simulink library "MATLAB_Function_lib"  (R2017b)
settings: Solver=VariableStepAuto  StartTime=0.0  StopTime=10.0  RelTol=1e-3
undefined symbols (not defined in the file or in its folder): Newton, Raphson
libraries: simulink x1
(part 1 of 3)
settings Model: Creator=ktrinh  LastModifiedBy=hbourbou

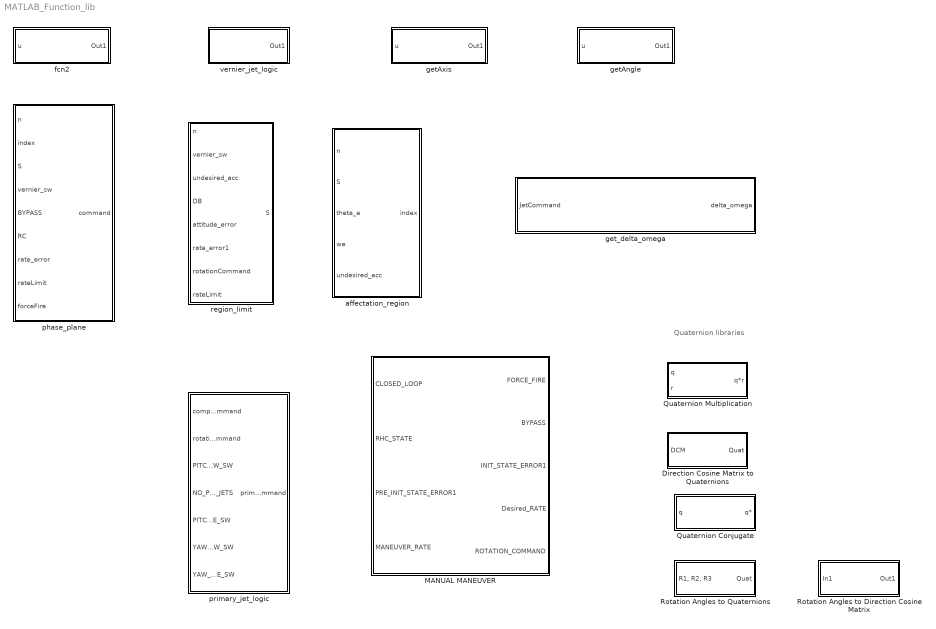
== system MATLAB_Function_lib ==
  note: Quaternion libraries
  Direction Cosine Matrix to Quaternions : Subsystem
  MANUAL MANEUVER : Subsystem
  Quaternion Conjugate : Subsystem
  Quaternion Multiplication : Subsystem
  Rotation Angles to Direction Cosine Matrix : Subsystem
  Rotation Angles to Quaternions : Subsystem
  affectation_region : Subsystem
  fcn2 : Subsystem
  getAngle : Subsystem
  getAxis : Subsystem
  get_delta_omega : Subsystem
  phase_plane : Subsystem
  primary_jet_logic : Subsystem
  region_limit : Subsystem
  vernier_jet_logic : Subsystem

== system MATLAB_Function_lib/Direction Cosine Matrix to Quaternions ==
  DCM : Inport  Unit=1  PortDimensions=[3,3]
  If : If
  Merge : Merge  InitialOutput=[1 0 0 0]
  Negative Trace : Subsystem
  Positive Trace : Subsystem  TreatAsAtomicUnit=on
  "Reshape 3x3 -> 9" : Reshape  OutputDimensions=[9,1]
  trace(DCM) : Subsystem
  Quat : Outport  Unit=1  PortDimensions=4
  wires:
  If/1 -> Positive Trace/Action
  Positive Trace/1(qw qx qy qz) -> Merge/1
  trace(DCM)/1(trace(DCM)) -> Positive Trace/1(trace(DCM)), If/1
  DCM/1 -> "Reshape 3x3 -> 9"/1
  "Reshape 3x3 -> 9"/1 -> trace(DCM)/1(DCM), Negative Trace/1(DCM), Positive Trace/2(DCM)
  Negative Trace/1(qw qx qy qz) -> Merge/2
  Merge/1 -> Quat/1
  If/2 -> Negative Trace/Action

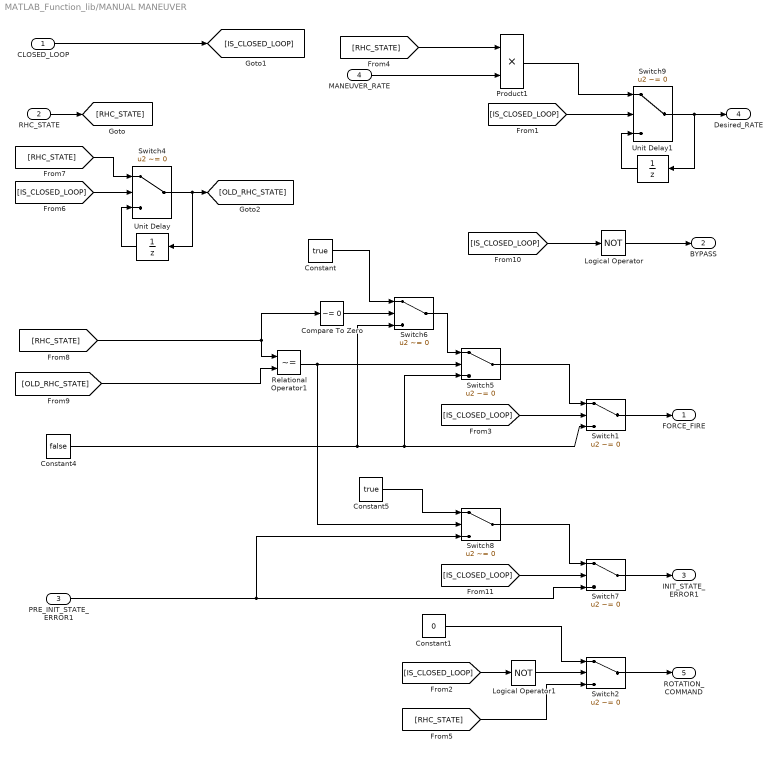
== system MATLAB_Function_lib/MANUAL MANEUVER ==
  CLOSED_LOOP : Inport
  RHC_STATE : Inport  Port=2
  PRE_INIT_STATE_ERROR1 : Inport  Port=3
  MANEUVER_RATE : Inport  Port=4
  Compare To Zero : simulink/Logic and Bit Operations/Compare To Zero  relop=~=  OutDataTypeStr=boolean
  Constant : Constant  Value=true
  Constant1 : Constant  Value=0
  Constant4 : Constant  Value=false
  Constant5 : Constant  Value=true
  Logical Operator : Logic  Operator=NOT  AllPortsSameDT=off  OutDataTypeStr=boolean
  Logical Operator1 : Logic  Operator=NOT  AllPortsSameDT=off  OutDataTypeStr=boolean
  Product1 : Product
  Relational Operator1 : RelationalOperator  Operator=~=  OutDataTypeStr=boolean  RndMeth=Simplest
  Switch{1..2,4..9} (8 alike) : Switch  Criteria=u2 ~= 0
  Unit Delay : UnitDelay  SampleTime=-1
  Unit Delay1 : UnitDelay  SampleTime=-1
  FORCE_FIRE : Outport
  BYPASS : Outport  Port=2
  INIT_STATE_ERROR1 : Outport  Port=3
  Desired_RATE : Outport  Port=4
  ROTATION_COMMAND : Outport  Port=5
  wires:
  Constant4/1 -> Switch6/3, Switch5/3, Switch1/3
  Switch1/1 -> FORCE_FIRE/1
  CLOSED_LOOP/1 -> [IS_CLOSED_LOOP]
  [IS_CLOSED_LOOP] -> Switch1/2
  RHC_STATE/1 -> [RHC_STATE]
  Switch4/1 -> Unit Delay/1, [OLD_RHC_STATE]
  [IS_CLOSED_LOOP] -> Switch4/2
  [RHC_STATE] -> Switch4/1
  Unit Delay/1 -> Switch4/3
  Switch5/1 -> Switch1/1
  [RHC_STATE] -> Compare To Zero/1, Relational Operator1/1
  [OLD_RHC_STATE] -> Relational Operator1/2
  Switch6/1 -> Switch5/1
  Compare To Zero/1 -> Switch6/2
  Constant/1 -> Switch6/1
  Logical Operator/1 -> BYPASS/1
  [IS_CLOSED_LOOP] -> Logical Operator/1
  Switch7/1 -> INIT_STATE_ERROR1/1
  Switch8/1 -> Switch7/1
  [IS_CLOSED_LOOP] -> Switch7/2
  Constant5/1 -> Switch8/1
  Relational Operator1/1 -> Switch8/2, Switch5/2
  PRE_INIT_STATE_ERROR1/1 -> Switch8/3, Switch7/3
  Switch9/1 -> Unit Delay1/1, Desired_RATE/1
  Product1/1 -> Switch9/1
  [IS_CLOSED_LOOP] -> Switch9/2
  [RHC_STATE] -> Product1/1
  MANEUVER_RATE/1 -> Product1/2
  Unit Delay1/1 -> Switch9/3
  [RHC_STATE] -> Switch2/3
  [IS_CLOSED_LOOP] -> Logical Operator1/1
  Constant1/1 -> Switch2/1
  Switch2/1 -> ROTATION_COMMAND/1
  Logical Operator1/1 -> Switch2/2

== system MATLAB_Function_lib/Quaternion Conjugate ==
  q : Inport  Unit=1
  Demux : Demux
  Mux : Mux
  Unary Minus : UnaryMinus
  Unary Minus1 : UnaryMinus
  Unary Minus2 : UnaryMinus
  q* : Outport  Unit=1
  wires:
  Mux/1 -> q*/1
  Demux/2 -> Unary Minus/1
  Unary Minus1/1 -> Mux/3
  Demux/4 -> Unary Minus2/1
  Demux/1 -> Mux/1
  Unary Minus/1 -> Mux/2
  Demux/3 -> Unary Minus1/1
  Unary Minus2/1 -> Mux/4
  q/1 -> Demux/1

== system MATLAB_Function_lib/Quaternion Multiplication ==
  q : Inport  Unit=1
  r : Inport  Port=2  Unit=1
  Mux : Mux
  q0 : Subsystem
  q1 : Subsystem
  q2 : Subsystem
  q3 : Subsystem
  q*r : Outport  Unit=1
  wires:
  q/1 -> q3/1(q), q2/1(q), q1/1(q), q0/1(q)
  q1/1(q1) -> Mux/2
  q0/1(q0) -> Mux/1
  q2/1(q2) -> Mux/3
  r/1 -> q3/2(r), q2/2(r), q1/2(r), q0/2(r)
  Mux/1 -> q*r/1
  q3/1(q3) -> Mux/4

== system MATLAB_Function_lib/Rotation Angles to Direction Cosine Matrix ==
  In1 : Inport  Unit=rad  PortDimensions=3
  Create 3x3 Matrix : Subsystem  mask(Create 3x3 Matrix){}
      mask help: shared_aeroblks:sharedaeroblkutil:blockCreate3x3MatrixDesc
      mask init:
      | if license('test','aerospace_blockset')
      |     aerosharedicon('shared');
      | elseif license('test','powertrain_blockset')
      |     sharedautoicon('shared');
      | end
      mask Help: eval('if license(''test'',''aerospace_blockset'')aerosharedhelp(''create_threebythree_matrix'');elseif license(''test'',''powertrain_blockset'')sharedautohelp(''create_threebythree_matrix'');end')
      mask Display:
      | port_label('input',1,'A_{11}','texmode','on');
      | port_label('input',2,'A_{12}','texmode','on');
      | port_label('input',3,'A_{13}','texmode','on');
      | port_label('input',4,'A_{21}','texmode','on');
      | port_label('input',5,'A_{22}','texmode','on');
      | port_label('input',6,'A_{23}','texmode','on');
      | port_label('input',7,'A_{31}','texmode','on');
      | port_label('input',8,'A_{32}','texmode','on');
      | port_label('input',9,'A_{33}','texmode','on');
      | port_label('output',1,'A','texmode','on');
  Fcn11 : Fcn  Expr=u(5)*u(6)
  Fcn12 : Fcn  Expr=u(1)*u(2)*u(6) + u(4)*u(3)
  Fcn13 : Fcn  Expr=-u(4)*u(2)*u(6) + u(1)*u(3)
  Fcn21 : Fcn  Expr=-u(5)*u(3)
  Fcn22 : Fcn  Expr=-u(1)*u(2)*u(3) + u(4)*u(6)
  Fcn23 : Fcn  Expr=u(4)*u(2)*u(3) + u(1)*u(6)
  Fcn31 : Fcn  Expr=u(2)
  Fcn32 : Fcn  Expr=-u(1)*u(5)
  Fcn33 : Fcn  Expr=u(4)*u(5)
  Mux : Mux  Inputs=2
  sincos : Trigonometry  Operator=sincos
  Out1 : Outport  Unit=1  PortDimensions=[3,3]
  wires:
  sincos/2 -> Mux/2
  Create 3x3 Matrix/1(Matrix) -> Out1/1
  Fcn11/1 -> Create 3x3 Matrix/1(M11)
  In1/1 -> sincos/1
  Fcn31/1 -> Create 3x3 Matrix/7(M31)
  Fcn22/1 -> Create 3x3 Matrix/5(M22)
  Fcn21/1 -> Create 3x3 Matrix/4(M21)
  Fcn23/1 -> Create 3x3 Matrix/6(M23)
  Fcn33/1 -> Create 3x3 Matrix/9(M33)
  Mux/1 -> Fcn11/1, Fcn12/1, Fcn13/1, Fcn21/1, Fcn32/1, Fcn33/1, Fcn31/1, Fcn23/1, Fcn22/1
  Fcn13/1 -> Create 3x3 Matrix/3(M13)
  sincos/1 -> Mux/1
  Fcn12/1 -> Create 3x3 Matrix/2(M12)
  Fcn32/1 -> Create 3x3 Matrix/8(M32)

== system MATLAB_Function_lib/Rotation Angles to Quaternions ==
  "R1, R2, R3" : Inport  Unit=rad
  1/2 : Gain  Gain=0.5  SaturateOnIntegerOverflow=on  OutDataTypeStr=Inherit: Same as input  ParamDataTypeStr=Inherit: Same as input
  Mux1 : Mux  Inputs=2
  Mux2 : Mux
  q0 : Fcn  Expr=u(4)*u(5)*u(6) - u(1)*u(2)*u(3)
  q1 : Fcn  Expr=u(4)*u(2)*u(3) + u(1)*u(5)*u(6)
  q2 : Fcn  Expr=u(4)*u(2)*u(6) - u(1)*u(5)*u(3)
  q3 : Fcn  Expr=u(4)*u(5)*u(3) + u(1)*u(2)*u(6)
  sincos : Trigonometry  Operator=sincos
  Quat : Outport  Unit=1  InitialOutput=0
  wires:
  q1/1 -> Mux2/2
  Mux2/1 -> Quat/1
  1/2/1 -> sincos/1
  sincos/1 -> Mux1/1
  q3/1 -> Mux2/4
  Mux1/1 -> q0/1, q1/1, q2/1, q3/1
  q0/1 -> Mux2/1
  "R1, R2, R3"/1 -> 1/2/1
  sincos/2 -> Mux1/2
  q2/1 -> Mux2/3

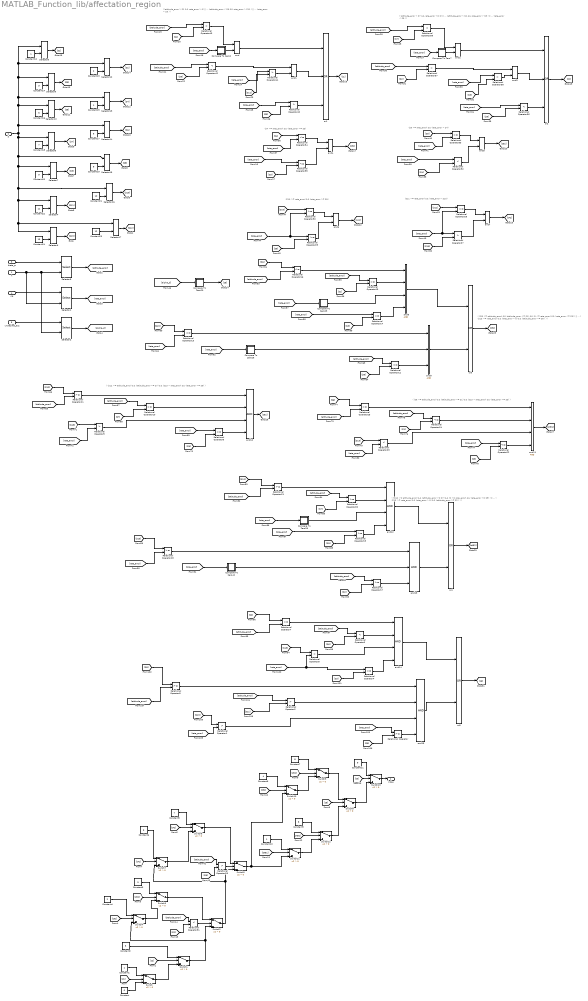
== system MATLAB_Function_lib/affectation_region ==
  note: ( (attitude_error > S1 && rate_error > 0) || ... (attitude_error < S8 && rate_error > S11 ) || ... (rate_error > S3 ) )
  note: ( (attitude_error < S7 && rate_error <= 0) || ... (attitude_error < S2 && rate_error > S5 ) || ... (rate_error < S9 ) )
  note: (S4 <= rate_error) && (rate_error <= S3)
  note: (S5 <= rate_error) && (rate_error < S4)
  note: (S10 >= rate_error) && (rate_error >= S9)
  note: (S11 >= rate_error) && (rate_error > S10)
  note: ( (S6 <= attitude_error) && (attitude_error <= S1) && (S13 < rate_error) && (rate_error <= S3) )
  note: ( ((S12 >= attitude_error) && (attitude_error >= S7) && (0 >= rate_error) && (rate_error >= S9) ) || ... ( (S13 >= rate_error) && (rate_error > 0) && (attitude_error >= S2 ) ) )
  note: ( (S12 >= attitude_error) && (attitude_error >= S7) && (S13 > rate_error) && (rate_error >= S9) )
  note: ( ((S6 <= attitude_error) && (attitude_error <= S1) && (0 <= rate_error) && (rate_error <= S3) ) || ... ( (S13 <= rate_error) && (rate_error < 0) && (attitude_error <= S8 ) ) )
  n : Inport
  S : Inport  Port=2
  theta_e : Inport  Port=3
  we : Inport  Port=4
  undesired_acc : Inport  Port=5
  Compare To Zero2 : Subsystem  mask(Compare To Zero){relop=>, OutDataTypeStr=boolean, ZeroCross=on}
      mask prompts: relop "Simulink:masks:Operator_MP"; OutDataTypeStr "Simulink:masks:OutputDataType_MP"; ZeroCross "Simulink:masks:EnableZerocrossingDetection_MP"
      mask help: Simulink:masks:CompareToZero_MD
      mask init:
      | blkName = gcb;
      | 
      | if strcmp(get_param(gcbh,'OutDataTypeStr'),'boolean')
      | 	setValue = 'boolean';
      | else
      |     setValue = 'fixdt(0, 8)';
      | end
      | 
      | set_param([blkName,'/Compare'],'relop',relop, ...
      | 	'OutDataTypeStr', setValue, 'ZeroCross', ZeroCross);
      mask TypeOptions relop: == | ~= | < | <= | >= | >
      mask TypeOptions OutDataTypeStr: Simulink:masks:uint8 | Simulink:masks:boolean
      mask Callback ZeroCross: sl('zeroCrossEnable', gcbh);
      mask Display: disp([relop,' 0'])
  Compare To Zero20 : Subsystem  mask(Compare To Zero){relop=>=, OutDataTypeStr=boolean, ZeroCross=on}
      mask prompts: relop "Simulink:masks:Operator_MP"; OutDataTypeStr "Simulink:masks:OutputDataType_MP"; ZeroCross "Simulink:masks:EnableZerocrossingDetection_MP"
      mask help: Simulink:masks:CompareToZero_MD
      mask init: same as MATLAB_Function_lib/affectation_region/Compare To Zero2
      mask TypeOptions relop: == | ~= | < | <= | >= | >
      mask TypeOptions OutDataTypeStr: Simulink:masks:uint8 | Simulink:masks:boolean
      mask Callback ZeroCross: sl('zeroCrossEnable', gcbh);
      mask Display: disp([relop,' 0'])
  Compare To Zero23 : Subsystem  mask(Compare To Zero){relop=>=, OutDataTypeStr=boolean, ZeroCross=on}
      mask prompts: relop "Simulink:masks:Operator_MP"; OutDataTypeStr "Simulink:masks:OutputDataType_MP"; ZeroCross "Simulink:masks:EnableZerocrossingDetection_MP"
      mask help: Simulink:masks:CompareToZero_MD
      mask init: same as MATLAB_Function_lib/affectation_region/Compare To Zero2
      mask TypeOptions relop: == | ~= | < | <= | >= | >
      mask TypeOptions OutDataTypeStr: Simulink:masks:uint8 | Simulink:masks:boolean
      mask Callback ZeroCross: sl('zeroCrossEnable', gcbh);
      mask Display: disp([relop,' 0'])
  Compare To Zero26 : Subsystem  mask(Compare To Zero){relop=<, OutDataTypeStr=boolean, ZeroCross=on}
      mask prompts: relop "Simulink:masks:Operator_MP"; OutDataTypeStr "Simulink:masks:OutputDataType_MP"; ZeroCross "Simulink:masks:EnableZerocrossingDetection_MP"
      mask help: Simulink:masks:CompareToZero_MD
      mask init: same as MATLAB_Function_lib/affectation_region/Compare To Zero2
      mask TypeOptions relop: == | ~= | < | <= | >= | >
      mask TypeOptions OutDataTypeStr: Simulink:masks:uint8 | Simulink:masks:boolean
      mask Callback ZeroCross: sl('zeroCrossEnable', gcbh);
      mask Display: disp([relop,' 0'])
  Compare To Zero39 : Subsystem  mask(Compare To Zero){relop=<=, OutDataTypeStr=boolean, ZeroCross=on}
      mask prompts: relop "Simulink:masks:Operator_MP"; OutDataTypeStr "Simulink:masks:OutputDataType_MP"; ZeroCross "Simulink:masks:EnableZerocrossingDetection_MP"
      mask help: Simulink:masks:CompareToZero_MD
      mask init: same as MATLAB_Function_lib/affectation_region/Compare To Zero2
      mask TypeOptions relop: == | ~= | < | <= | >= | >
      mask TypeOptions OutDataTypeStr: Simulink:masks:uint8 | Simulink:masks:boolean
      mask Callback ZeroCross: sl('zeroCrossEnable', gcbh);
      mask Display: disp([relop,' 0'])
  Compare To Zero42 : Subsystem  mask(Compare To Zero){relop=>, OutDataTypeStr=boolean, ZeroCross=on}
      mask prompts: relop "Simulink:masks:Operator_MP"; OutDataTypeStr "Simulink:masks:OutputDataType_MP"; ZeroCross "Simulink:masks:EnableZerocrossingDetection_MP"
      mask help: Simulink:masks:CompareToZero_MD
      mask init: same as MATLAB_Function_lib/affectation_region/Compare To Zero2
      mask TypeOptions relop: == | ~= | < | <= | >= | >
      mask TypeOptions OutDataTypeStr: Simulink:masks:uint8 | Simulink:masks:boolean
      mask Callback ZeroCross: sl('zeroCrossEnable', gcbh);
      mask Display: disp([relop,' 0'])
  Compare To Zero7 : Subsystem  mask(Compare To Zero){relop=<=, OutDataTypeStr=boolean, ZeroCross=on}
      mask prompts: relop "Simulink:masks:Operator_MP"; OutDataTypeStr "Simulink:masks:OutputDataType_MP"; ZeroCross "Simulink:masks:EnableZerocrossingDetection_MP"
      mask help: Simulink:masks:CompareToZero_MD
      mask init: same as MATLAB_Function_lib/affectation_region/Compare To Zero2
      mask TypeOptions relop: == | ~= | < | <= | >= | >
      mask TypeOptions OutDataTypeStr: Simulink:masks:uint8 | Simulink:masks:boolean
      mask Callback ZeroCross: sl('zeroCrossEnable', gcbh);
      mask Display: disp([relop,' 0'])
  Constant : Constant  Value=0
  Constant1 : Constant
  Constant10 : Constant  Value=4
  Constant11 : Constant  Value=9
  Constant12 : Constant
  Constant13 : Constant  Value=2
  Constant14 : Constant  Value=3
  Constant15 : Constant  Value=4
  Constant16 : Constant  Value=5
  Constant17 : Constant  Value=6
  Constant18 : Constant  Value=7
  Constant19 : Constant  Value=8
  Constant2 : Constant  Value=5
  Constant20 : Constant  Value=9
  Constant21 : Constant  Value=10
  Constant22 : Constant  Value=11
  Constant23 : Constant  Value=12
  Constant24 : Constant  Value=13
  Constant3 : Constant  Value=3
  Constant4 : Constant  Value=2
  Constant5 : Constant  Value=7
  Constant6 : Constant  Value=6
  Constant7 : Constant  Value=8
  Constant8 : Constant  Value=4
  Constant9 : Constant  Value=8
  Relational Operator{,3,8,10..11,17..21,28..30} (13 alike) : RelationalOperator  OutDataTypeStr=boolean  RndMeth=Simplest
  Relational Operator{1..2,9,26..27,38,40..41,43} (9 alike) : RelationalOperator  Operator=>  OutDataTypeStr=boolean  RndMeth=Simplest
  Relational Operator{4,7,12..16,22,24..25,33..35} (13 alike) : RelationalOperator  Operator=<=  OutDataTypeStr=boolean  RndMeth=Simplest
  Relational Operator{5..6,23,31..32,36..37,39,42} (9 alike) : RelationalOperator  Operator=<  OutDataTypeStr=boolean  RndMeth=Simplest
  Selector1 : Selector  InputPortWidth=3  IndexOptions=Index vector (port)  Indices=[1 3]  OutputSizes=1
  Selector{3..4,6..10,12..17} (13 alike) : Selector  InputPortWidth=13  IndexOptions=Starting index (port)  Indices=[1 3]  OutputSizes=1
  Selector2 : Selector  InputPortWidth=3  IndexOptions=Index vector (port)  Indices=[1 3]  OutputSizes=1
  Selector5 : Selector  InputPortWidth=3  IndexOptions=Index vector (port)  Indices=[1 3]  OutputSizes=1
  Switch{,1..13} (14 alike) : Switch  Criteria=u2 > Threshold
  and{,1..7} (8 alike) : Logic  AllPortsSameDT=off  OutDataTypeStr=boolean
  and{8,10..12,14..15} (6 alike) : Logic  Inputs=4  AllPortsSameDT=off  OutDataTypeStr=boolean
  and13 : Logic  Inputs=3  AllPortsSameDT=off  OutDataTypeStr=boolean
  and9 : Logic  Inputs=3  AllPortsSameDT=off  OutDataTypeStr=boolean
  or1 : Logic  Operator=OR  Inputs=3  AllPortsSameDT=off  OutDataTypeStr=boolean
  or2 : Logic  Operator=OR  Inputs=3  AllPortsSameDT=off  OutDataTypeStr=boolean
  or3 : Logic  Operator=OR  AllPortsSameDT=off  OutDataTypeStr=boolean
  or4 : Logic  Operator=OR  AllPortsSameDT=off  OutDataTypeStr=boolean
  or5 : Logic  Operator=OR  AllPortsSameDT=off  OutDataTypeStr=boolean
  index : Outport
  wires:
  theta_e/1 -> Selector5/1
  we/1 -> Selector1/1
  Selector5/1 -> [attitude_error]
  Selector1/1 -> [rate_error]
  Selector2/1 -> [alpha_d]
  undesired_acc/1 -> Selector2/1
  n/1 -> Selector1/2, Selector2/2, Selector5/2
  Selector10/1 -> [S5]
  Selector13/1 -> [S4]
  Selector12/1 -> [S2]
  Constant/1 -> Switch/3
  Switch/1 -> Switch1/3
  Constant1/1 -> Switch/1
  [c1] -> Switch/2
  [c2] -> Switch1/2
  Constant2/1 -> Switch1/1
  Switch1/1 -> Switch4/3, Switch2/3
  Relational Operator31/1 -> Switch2/2
  Switch3/1 -> Switch2/1
  Switch4/1 -> Switch3/3
  [c32] -> Switch3/2
  Constant3/1 -> Switch3/1
  [c31] -> Switch4/2
  Constant4/1 -> Switch4/1
  Relational Operator26/1 -> Switch5/2
  Switch2/1 -> Switch5/3, Switch7/3
  Switch7/1 -> Switch6/3
  [c42] -> Switch6/2
  Constant6/1 -> Switch7/1
  Constant5/1 -> Switch6/1
  Switch6/1 -> Switch5/1
  [c41] -> Switch7/2
  [c5] -> Switch8/2
  [c52] -> Switch9/2
  Constant7/1 -> Switch9/1
  Switch10/1 -> Switch9/3
  [c51] -> Switch10/2
  Constant8/1 -> Switch10/1
  Switch9/1 -> Switch8/1
  Switch11/1 -> Switch12/3
  Switch12/1 -> Switch8/3
  Constant9/1 -> Switch12/1
  Switch5/1 -> Switch11/3, Switch10/3
  [cN51] -> Switch11/2
  Constant10/1 -> Switch11/1
  [cN52] -> Switch12/2
  [c6] -> Switch13/2
  Constant11/1 -> Switch13/1
  Switch8/1 -> Switch13/3
  Switch13/1 -> index/1
  Selector3/1 -> [S1]
  Constant12/1 -> Selector3/2
  Constant13/1 -> Selector12/2
  Constant14/1 -> Selector9/2
  Constant15/1 -> Selector13/2
  Constant16/1 -> Selector10/2
  Constant17/1 -> Selector14/2
  Selector14/1 -> [S6]
  Constant18/1 -> Selector8/2
  Selector8/1 -> [S7]
  Selector15/1 -> [S8]
  Constant19/1 -> Selector15/2
  Selector7/1 -> [S9]
  Constant20/1 -> Selector7/2
  Constant21/1 -> Selector16/2
  Selector16/1 -> [S10]
  Constant22/1 -> Selector4/2
  Selector4/1 -> [S11]
  S/1 -> Selector8/1, Selector15/1, Selector7/1, Selector16/1, Selector4/1, Selector6/1, Selector17/1, Selector14/1, Selector10/1, Selector13/1, Selector9/1, Selector12/1, Selector3/1
  Constant23/1 -> Selector17/2
  Selector17/1 -> [S12]
  Constant24/1 -> Selector6/2
  Selector6/1 -> [S13]
  or1/1 -> [c1]
  and/1 -> or1/1
  [rate_error] -> Compare To Zero2/1(u)
  Compare To Zero2/1(y) -> and/2
  Relational Operator43/1 -> and/1
  [attitude_error] -> Relational Operator43/1
  [S1] -> Relational Operator43/2
  [S8] -> Relational Operator42/2
  [attitude_error] -> Relational Operator42/1
  Relational Operator42/1 -> and1/1
  and1/1 -> or1/2
  Relational Operator41/1 -> and1/2
  [S11] -> Relational Operator41/2
  [rate_error] -> Relational Operator41/1
  Relational Operator40/1 -> or1/3
  [S3] -> Relational Operator40/2
  Relational Operator39/1 -> and2/1
  [rate_error] -> Relational Operator38/1
  Relational Operator37/1 -> and3/1
  [S7] -> Relational Operator39/2
  and3/1 -> or2/2
  [attitude_error] -> Relational Operator39/1
  Relational Operator38/1 -> and3/2
  Relational Operator36/1 -> or2/3
  [S2] -> Relational Operator37/2
  or2/1 -> [c2]
  [S9] -> Relational Operator36/2
  and2/1 -> or2/1
  [S5] -> Relational Operator38/2
  Compare To Zero7/1(y) -> and2/2
  [rate_error] -> Relational Operator36/1
  [rate_error] -> Compare To Zero7/1(u)
  and4/1 -> [c31]
  [rate_error] -> Relational Operator35/1
  [S3] -> Relational Operator35/2
  [S4] -> Relational Operator34/1
  Relational Operator34/1 -> and4/1
  Relational Operator35/1 -> and4/2
  [rate_error] -> Relational Operator33/2
  [S4] -> Relational Operator32/2
  Relational Operator32/1 -> and5/2
  [S5] -> Relational Operator33/1
  and5/1 -> [c32]
  Relational Operator33/1 -> and5/1
  [rate_error] -> Relational Operator32/1
  [rate_error] -> Relational Operator28/2, Relational Operator27/1
  Relational Operator28/1 -> and7/1
  and7/1 -> [c42]
  Relational Operator27/1 -> and7/2
  [S9] -> Relational Operator29/2
  Relational Operator29/1 -> and6/2
  [S10] -> Relational Operator27/2
  Relational Operator30/1 -> and6/1
  [S10] -> Relational Operator30/1
  [S11] -> Relational Operator28/1
  and6/1 -> [c41]
  [rate_error] -> Relational Operator30/2, Relational Operator29/1
  Compare To Zero20/1(y) -> [c5]
  [alpha_d] -> Compare To Zero20/1(u)
  or3/1 -> [c51]
  and8/1 -> or3/1
  and9/1 -> or3/2
  Relational Operator16/1 -> and8/1
  [S6] -> Relational Operator16/1
  [attitude_error] -> Relational Operator16/2
  Relational Operator15/1 -> and8/2
  [attitude_error] -> Relational Operator15/1
  [S1] -> Relational Operator15/2
  [rate_error] -> Compare To Zero23/1(u)
  Compare To Zero23/1(y) -> and8/3
  [rate_error] -> Relational Operator14/1
  Relational Operator14/1 -> and8/4
  [S3] -> Relational Operator14/2
  [rate_error] -> Relational Operator13/2
  Relational Operator13/1 -> and9/1
  [S13] -> Relational Operator13/1
  Compare To Zero26/1(y) -> and9/2
  [rate_error] -> Compare To Zero26/1(u)
  Relational Operator12/1 -> and9/3
  [attitude_error] -> Relational Operator12/1
  [S8] -> Relational Operator12/2
  and10/1 -> [c52]
  Relational Operator11/1 -> and10/1
  [attitude_error] -> Relational Operator11/2
  Relational Operator10/1 -> and10/2
  [attitude_error] -> Relational Operator10/1
  [S7] -> Relational Operator10/2
  Relational Operator8/1 -> and10/4
  [S9] -> Relational Operator8/2
  [rate_error] -> Relational Operator8/1
  Relational Operator9/1 -> and10/3
  [rate_error] -> Relational Operator9/2
  [S13] -> Relational Operator9/1
  and11/1 -> [cN51]
  Relational Operator24/1 -> and11/2
  [attitude_error] -> Relational Operator25/2
  [S13] -> Relational Operator23/1
  [S3] -> Relational Operator22/2
  Relational Operator22/1 -> and11/4
  Relational Operator25/1 -> and11/1
  Relational Operator23/1 -> and11/3
  [S6] -> Relational Operator25/1
  [rate_error] -> Relational Operator23/2
  [rate_error] -> Relational Operator22/1
  [S1] -> Relational Operator24/2
  Compare To Zero39/1(y) -> and12/3
  Relational Operator21/1 -> and12/1
  [attitude_error] -> Relational Operator21/2
  [rate_error] -> Compare To Zero39/1(u)
  [attitude_error] -> Relational Operator17/1
  [S2] -> Relational Operator17/2
  [attitude_error] -> Relational Operator20/1
  Relational Operator17/1 -> and13/3
  Relational Operator20/1 -> and12/2
  or4/1 -> [cN52]
  Relational Operator19/1 -> and12/4
  [rate_error] -> Relational Operator19/1
  [rate_error] -> Relational Operator18/2
  Relational Operator18/1 -> and13/1
  [rate_error] -> Compare To Zero42/1(u)
  [S9] -> Relational Operator19/2
  and13/1 -> or4/2
  [S12] -> Relational Operator21/1
  [S13] -> Relational Operator18/1
  and12/1 -> or4/1
  Compare To Zero42/1(y) -> and13/2
  [S7] -> Relational Operator20/2
  [S2] -> Relational Operator7/1
  Relational Operator7/1 -> and14/1
  [attitude_error] -> Relational Operator7/2
  [rate_error] -> Relational Operator5/2, Relational Operator4/1
  and15/1 -> or5/2
  [S6] -> Relational Operator6/2
  [attitude_error] -> Relational Operator6/1
  and14/1 -> or5/1
  or5/1 -> [c6]
  [rate_error] -> Relational Operator/1
  Relational Operator6/1 -> and14/2
  Relational Operator2/1 -> and15/2
  [S9] -> Relational Operator/2
  Relational Operator3/1 -> and15/1
  Relational Operator5/1 -> and14/3
  [S3] -> Relational Operator4/2
  Relational Operator4/1 -> and14/4
  [S13] -> Relational Operator5/1
  [attitude_error] -> Relational Operator3/2
  [S8] -> Relational Operator3/1
  [S12] -> Relational Operator2/2
  [attitude_error] -> Relational Operator2/1
  Relational Operator/1 -> and15/4
  Relational Operator1/1 -> and15/3
  [S13] -> Relational Operator1/1
  Selector9/1 -> [S3]
  [rate_error] -> Relational Operator1/2
  [S12] -> Relational Operator11/1
  [attitude_error] -> Relational Operator24/1
  [S8] -> Relational Operator26/2
  [attitude_error] -> Relational Operator26/1
  [S2] -> Relational Operator31/2
  [attitude_error] -> Relational Operator31/1
  [rate_error] -> Relational Operator34/2
  [attitude_error] -> Relational Operator37/1
  [rate_error] -> Relational Operator40/1

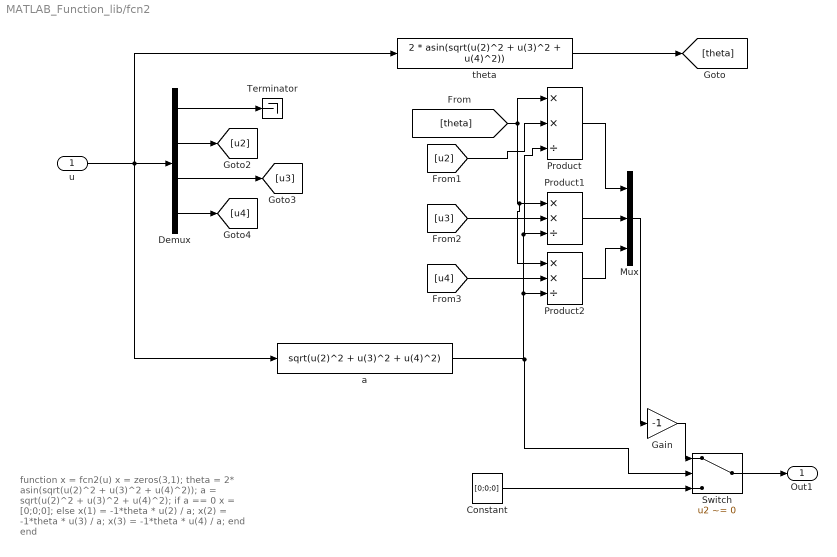
== system MATLAB_Function_lib/fcn2 ==
  note: function x = fcn2(u)
      |
      | x = zeros(3,1);
      |
      | theta = 2* asin(sqrt(u(2)^2 + u(3)^2 + u(4)^2));
      |
      | a = sqrt(u(2)^2 + u(3)^2 + u(4)^2);
      |
      | if a == 0
      |
      | x = [0;0;0];
      |
      | else
      |
      | x(1) = -1*theta * u(2) / a;
      |
      | x(2) = -1*theta * u(3) / a;
      |
      | x(3) = -1*theta * u(4) / a;
      |
      | end
      |
      | end
  u : Inport
  Constant : Constant  Value=[0;0;0]
  Demux : Demux
  Gain : Gain  Gain=-1
  Mux : Mux  Inputs=3
  Product : Product  Inputs=**/
  Product1 : Product  Inputs=**/
  Product2 : Product  Inputs=**/
  Switch : Switch  Criteria=u2 ~= 0
  Terminator : Terminator
  a : Fcn  Expr=sqrt(u(2)^2 + u(3)^2 + u(4)^2)
  theta : Fcn  Expr=2 * asin(sqrt(u(2)^2 + u(3)^2 + u(4)^2))
  Out1 : Outport
  wires:
  u/1 -> a/1, Demux/1, theta/1
  Constant/1 -> Switch/3
  Switch/1 -> Out1/1
  Demux/1 -> Terminator/1
  theta/1 -> [theta]
  Product/1 -> Mux/1
  [theta] -> Product2/1, Product1/1, Product/1
  Demux/2 -> [u2]
  Demux/3 -> [u3]
  Demux/4 -> [u4]
  [u2] -> Product/2
  [u3] -> Product1/2
  Product1/1 -> Mux/2
  Product2/1 -> Mux/3
  [u4] -> Product2/2
  a/1 -> Switch/2, Product2/3, Product/3, Product1/3
  Mux/1 -> Gain/1
  Gain/1 -> Switch/1

== system MATLAB_Function_lib/getAngle ==
  u : Inport
  theta : Fcn  Expr=2*asin(sqrt( u(2)^2 + u(3)^2 + u(4)^2 ) )
  Out1 : Outport
  wires:
  theta/1 -> Out1/1
  u/1 -> theta/1

== system MATLAB_Function_lib/getAxis ==
  u : Inport
  Constant : Constant  Value=[1;0;0]
  Demux : Demux
  Gain1 : Gain  Gain=-1
  Mux : Mux  Inputs=3
  Product1 : Product  Inputs=*/
  Product2 : Product  Inputs=*/
  Product3 : Product  Inputs=*/
  Switch : Switch  Criteria=u2 > Threshold
  Terminator : Terminator
  a : Fcn  Expr=sqrt(u(2)^2 + u(3)^2 + u(4)^2)
  Out1 : Outport
  wires:
  Switch/1 -> Out1/1
  Constant/1 -> Switch/3
  a/1 -> Product2/2, Product1/2, Product3/2, Switch/2
  u/1 -> Demux/1, a/1
  Demux/1 -> Terminator/1
  Demux/2 -> Product3/1
  Product3/1 -> Mux/1
  Product2/1 -> Mux/3
  Product1/1 -> Mux/2
  Demux/3 -> Product1/1
  Demux/4 -> Product2/1
  Mux/1 -> Gain1/1
  Gain1/1 -> Switch/1

== system MATLAB_Function_lib/get_delta_omega ==
  JetCommand : Inport
  Constant : Constant  Value="[   0       -0.03389  0       ; -0.01775  0.02513 -0.02364 ; 0.01778  0.02514  0.02363 ;      -0.03573  0.01901 -0.00293 ;    0.03607  0.01904  0.00294 ;      0.02849 -0.01281 -0.00458 ;      -0.02876 -0.01284  0.00457 ;     0.00547 -0.00037  0.03194 ;     -0.00547 -0.00036 -0.03194 ;    0.02112   0       -0.01763 ;       -0.02113   0        0.01763 ;            -0.0004152  0.0007067 -0.0006653  ;    0.0004162  0.0007069  0.0006652  ;    -0.0006727 -0.0000146  0.0005203  ;    0.0006724 -0.0000138 -0.0005203  ;  -0.0005994 -0.0003125 -0.0000201  ; 0.0005942 -0.0003120 0.0000200]"
  For Iterator Subsystem : Subsystem  TreatAsAtomicUnit=on
  delta_omega : Outport
  wires:
  Constant/1 -> For Iterator Subsystem/2(matrix_delta_omega_jet)
  For Iterator Subsystem/1(Out1) -> delta_omega/1
  JetCommand/1 -> For Iterator Subsystem/1(JetCommand)

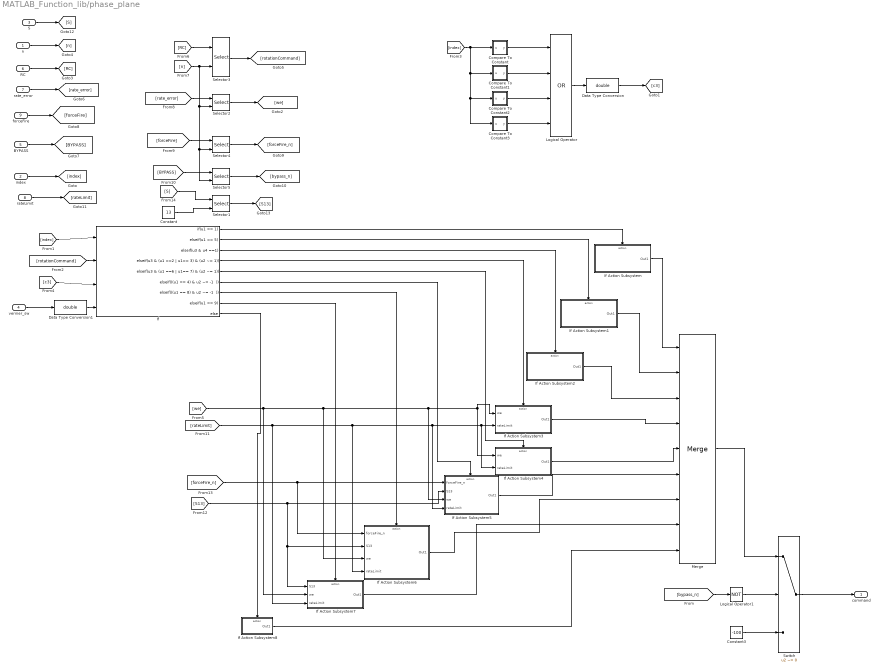
== system MATLAB_Function_lib/phase_plane ==
  n : Inport
  index : Inport  Port=2  OutDataTypeStr=double
  S : Inport  Port=3
  vernier_sw : Inport  Port=4
  BYPASS : Inport  Port=5
  RC : Inport  Port=6
  rate_error : Inport  Port=7
  rateLimit : Inport  Port=8
  forceFire : Inport  Port=9  OutDataTypeStr=boolean  PortDimensions=3
  Compare To Constant : Subsystem  mask(Compare To Constant){relop===, const=2, OutDataTypeStr=boolean, ZeroCross=on}
      mask prompts: relop "Simulink:masks:Operator_MP"; const "Simulink:masks:ConstantValue_MP"; OutDataTypeStr "Simulink:masks:OutputDataType_MP"; ZeroCross "Simulink:masks:EnableZerocrossingDetection_MP"
      mask help: Simulink:masks:CompareToConstant_MD
      mask init:
      | blkName = gcb;
      | 
      | if strcmp(get_param(gcbh,'OutDataTypeStr'),'boolean')
      | 	setValue = 'boolean';
      | else
      | 	setValue = 'fixdt(0, 8)';
      | end
      | 
      | set_param([blkName,'/Compare'],'relop',relop, ...
      | 	'OutDataTypeStr', setValue, 'ZeroCross', ZeroCross);
      | 
      | str = [relop,' C']; %default
      | 
      | const_str = get_param(blkName, 'const');
      | const_val = str2num(const_str);
      | 
      | if isempty(const_val) %#ok<ST2NM>
      |     %Expression/Variable
      |     str = [relop, ' ', strtrim(const_str)];
      | else
      |     if length(const_val) == 1 
      |         if Simulink.data.isSupportedEnumClass(class(const_val))
      |             % Special Handling for Enumerations
      |             if Simulink.data.getEnumTypeInfo(class(const_val), 'AddClassNameToEnumNames')
      |                 str = [relop, ' ', strtrim(const_str)];
      |             else
      |                 str = [relop, ' ', char(const_val)];
      |             end
      |         elseif(isfloat(const_val) || isinteger(const_val) || islogical(const_val)) 
      |                 str = [relop, ' ', num2str(const_val)];
      |         end
      |     end
      | end
      mask TypeOptions relop: == | ~= | < | <= | >= | >
      mask TypeOptions OutDataTypeStr: Simulink:masks:uint8 | Simulink:masks:boolean
      mask Callback ZeroCross: sl('zeroCrossEnable', gcbh);
      mask Display: disp(str)
  Compare To Constant1 : Subsystem  mask(Compare To Constant){relop===, const=3, OutDataTypeStr=boolean, ZeroCross=on}
      mask prompts: relop "Simulink:masks:Operator_MP"; const "Simulink:masks:ConstantValue_MP"; OutDataTypeStr "Simulink:masks:OutputDataType_MP"; ZeroCross "Simulink:masks:EnableZerocrossingDetection_MP"
      mask help: Simulink:masks:CompareToConstant_MD
      mask init: same as MATLAB_Function_lib/phase_plane/Compare To Constant
      mask TypeOptions relop: == | ~= | < | <= | >= | >
      mask TypeOptions OutDataTypeStr: Simulink:masks:uint8 | Simulink:masks:boolean
      mask Callback ZeroCross: sl('zeroCrossEnable', gcbh);
      mask Display: disp(str)
  Compare To Constant2 : Subsystem  mask(Compare To Constant){relop===, const=6, OutDataTypeStr=boolean, ZeroCross=on}
      mask prompts: relop "Simulink:masks:Operator_MP"; const "Simulink:masks:ConstantValue_MP"; OutDataTypeStr "Simulink:masks:OutputDataType_MP"; ZeroCross "Simulink:masks:EnableZerocrossingDetection_MP"
      mask help: Simulink:masks:CompareToConstant_MD
      mask init: same as MATLAB_Function_lib/phase_plane/Compare To Constant
      mask TypeOptions relop: == | ~= | < | <= | >= | >
      mask TypeOptions OutDataTypeStr: Simulink:masks:uint8 | Simulink:masks:boolean
      mask Callback ZeroCross: sl('zeroCrossEnable', gcbh);
      mask Display: disp(str)
  Compare To Constant3 : Subsystem  mask(Compare To Constant){relop===, const=7, OutDataTypeStr=boolean, ZeroCross=on}
      mask prompts: relop "Simulink:masks:Operator_MP"; const "Simulink:masks:ConstantValue_MP"; OutDataTypeStr "Simulink:masks:OutputDataType_MP"; ZeroCross "Simulink:masks:EnableZerocrossingDetection_MP"
      mask help: Simulink:masks:CompareToConstant_MD
      mask init: same as MATLAB_Function_lib/phase_plane/Compare To Constant
      mask TypeOptions relop: == | ~= | < | <= | >= | >
      mask TypeOptions OutDataTypeStr: Simulink:masks:uint8 | Simulink:masks:boolean
      mask Callback ZeroCross: sl('zeroCrossEnable', gcbh);
      mask Display: disp(str)
  Constant : Constant  Value=13
  Constant3 : Constant  Value=-100
  Data Type Conversion : DataTypeConversion  OutDataTypeStr=double
  Data Type Conversion1 : DataTypeConversion  OutDataTypeStr=double
  If : If  NumInputs=4  IfExpression=u1 == 1  ElseIfExpressions="u1 == 5, u3 & u4 ==1, u3 & (u1 ==2 | u1== 3) & (u2 ~= 1), u3 & (u1 ==6 | u1== 7) & (u2 ~= 1), ((u1 == 4) & u2 ~= -1  ), ((u1 == 8) & u2 ~= -1  ), u1 == 9"
  If Action Subsystem : Subsystem  TreatAsAtomicUnit=on
  If Action Subsystem1 : Subsystem  TreatAsAtomicUnit=on
  If Action Subsystem2 : Subsystem  TreatAsAtomicUnit=on
  If Action Subsystem3 : Subsystem  TreatAsAtomicUnit=on
  If Action Subsystem4 : Subsystem  TreatAsAtomicUnit=on
  If Action Subsystem5 : Subsystem  TreatAsAtomicUnit=on
  If Action Subsystem6 : Subsystem  TreatAsAtomicUnit=on
  If Action Subsystem7 : Subsystem  TreatAsAtomicUnit=on
  If Action Subsystem8 : Subsystem  TreatAsAtomicUnit=on
  Logical Operator : Logic  Operator=OR  Inputs=4  AllPortsSameDT=off  OutDataTypeStr=fixdt(1,16)
  Logical Operator1 : Logic  Operator=NOT  AllPortsSameDT=off  OutDataTypeStr=boolean
  Merge : Merge  Inputs=9
  Selector1 : Selector  InputPortWidth=13  IndexOptions=Index vector (port)  Indices=[1 3]  OutputSizes=1
  Selector{2..5} (4 alike) : Selector  InputPortWidth=3  IndexOptions=Index vector (port)  Indices=[1 3]  OutputSizes=1
  Switch : Switch  Criteria=u2 ~= 0
  command : Outport
  wires:
  RC/1 -> [RC]
  n/1 -> [n]
  [RC] -> Selector3/1
  Selector3/1 -> [rotationCommand]
  rate_error/1 -> [rate_error]
  [rate_error] -> Selector2/1
  [n] -> Selector5/2, Selector4/2, Selector2/2, Selector3/2
  Selector2/1 -> [we]
  BYPASS/1 -> [BYPASS]
  forceFire/1 -> [forceFire]
  Selector4/1 -> [forceFire_n]
  [forceFire] -> Selector4/1
  Selector5/1 -> [bypass_n]
  [BYPASS] -> Selector5/1
  Constant3/1 -> Switch/3
  Switch/1 -> command/1
  Logical Operator1/1 -> Switch/2
  [bypass_n] -> Logical Operator1/1
  index/1 -> [index]
  [index] -> If/1
  [rotationCommand] -> If/2
  If/1 -> If Action Subsystem/Action
  If/2 -> If Action Subsystem1/Action
  If/3 -> If Action Subsystem2/Action
  If/4 -> If Action Subsystem3/Action
  If/5 -> If Action Subsystem4/Action
  If/6 -> If Action Subsystem5/Action
  If Action Subsystem/1(Out1) -> Merge/1
  If Action Subsystem1/1(Out1) -> Merge/2
  If Action Subsystem2/1(Out1) -> Merge/3
  If Action Subsystem3/1(Out1) -> Merge/4
  If Action Subsystem4/1(Out1) -> Merge/5
  If Action Subsystem5/1(Out1) -> Merge/6
  Merge/1 -> Switch/1
  Logical Operator/1 -> Data Type Conversion/1
  Compare To Constant/1(y) -> Logical Operator/1
  [index] -> Compare To Constant3/1(u), Compare To Constant2/1(u), Compare To Constant1/1(u), Compare To Constant/1(u)
  Compare To Constant1/1(y) -> Logical Operator/2
  Compare To Constant2/1(y) -> Logical Operator/3
  Compare To Constant3/1(y) -> Logical Operator/4
  [c3] -> If/3
  vernier_sw/1 -> Data Type Conversion1/1
  If/7 -> If Action Subsystem6/Action
  If/8 -> If Action Subsystem7/Action
  If Action Subsystem6/1(Out1) -> Merge/7
  If Action Subsystem7/1(Out1) -> Merge/8
  [we] -> If Action Subsystem7/2(we), If Action Subsystem6/3(we), If Action Subsystem5/3(we), If Action Subsystem3/1(we), If Action Subsystem4/1(we)
  [rateLimit] -> If Action Subsystem7/3(rateLimit), If Action Subsystem6/4(rateLimit), If Action Subsystem5/4(rateLimit), If Action Subsystem4/2(rateLimit), If Action Subsystem3/2(rateLimit)
  rateLimit/1 -> [rateLimit]
  [S13] -> If Action Subsystem7/1(S13), If Action Subsystem6/2(S13), If Action Subsystem5/2(S13)
  [forceFire_n] -> If Action Subsystem6/1(forceFire_n), If Action Subsystem5/1(forceFire_n)
  S/1 -> [S]
  [S] -> Selector1/1
  Constant/1 -> Selector1/2
  Selector1/1 -> [S13]
  Data Type Conversion/1 -> [c3]
  If/9 -> If Action Subsystem8/Action
  If Action Subsystem8/1(Out1) -> Merge/9
  Data Type Conversion1/1 -> If/4

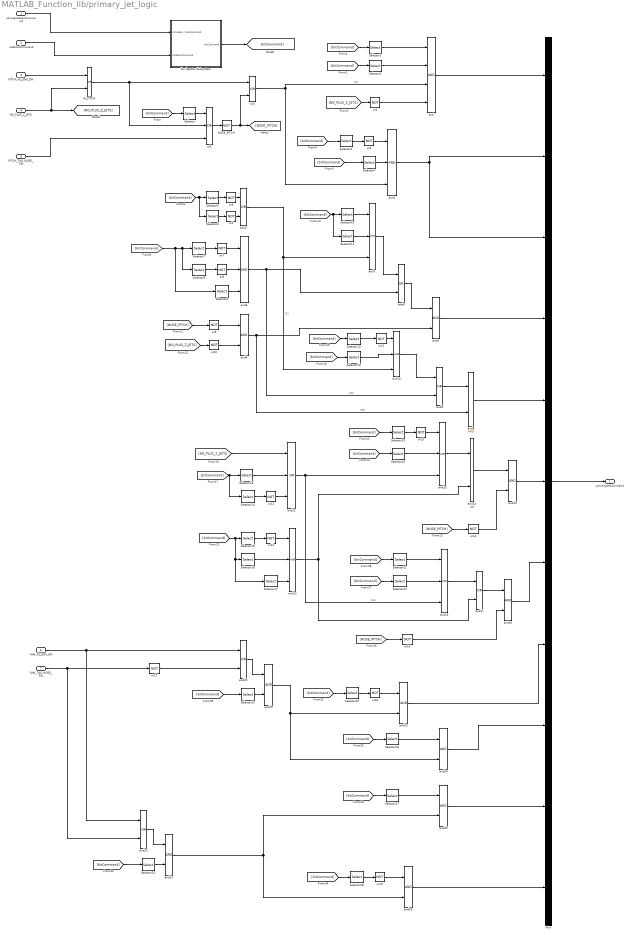
== system MATLAB_Function_lib/primary_jet_logic ==
  compensationCommand : Inport
  rotationCommand : Inport  Port=2
  PITCH_HI_LOW_SW : Inport  Port=3
  NO_PLUS_Z_JETS : Inport  Port=4
  PITCH_TAIL_NOSE_SW : Inport  Port=5
  YAW_HI_LOW_SW : Inport  Port=6
  YAW_TAIL_NOSE_SW : Inport  Port=7
  For Iterator Subsystem : Subsystem  TreatAsAtomicUnit=on
  HI_PITCH : Logic  Operator=OR  AllPortsSameDT=off  OutDataTypeStr=boolean
  Mux : Mux  Inputs=11
  NOSE_PITCH : Logic  Operator=NOT  Inputs=1  AllPortsSameDT=off  OutDataTypeStr=boolean
  Selector{,7,11,13,15,20,22} (7 alike) : Selector  InputPortWidth=6  IndexOptions=Index vector (dialog)  Indices=[2]  OutputSizes=1
  Selector{1,3,5,9,16,18} (6 alike) : Selector  InputPortWidth=6  IndexOptions=Index vector (dialog)  Indices=[3]  OutputSizes=1
  Selector{10,12,19,21} (4 alike) : Selector  InputPortWidth=6  IndexOptions=Index vector (dialog)  Indices=[1]  OutputSizes=1
  Selector{2,4,6,8,14,17} (6 alike) : Selector  InputPortWidth=6  IndexOptions=Index vector (dialog)  Indices=[4]  OutputSizes=1
  Selector23 : Selector  InputPortWidth=6  IndexOptions=Index vector (dialog)  Indices=[6]  OutputSizes=1
  Selector24 : Selector  InputPortWidth=6  IndexOptions=Index vector (dialog)  Indices=[6]  OutputSizes=1
  Selector{25..28} (4 alike) : Selector  InputPortWidth=6  IndexOptions=Index vector (dialog)  Indices=[5]  OutputSizes=1
  and : Logic  Inputs=4  AllPortsSameDT=off  OutDataTypeStr=boolean
  and{1,3,7,10,12,15,18} (7 alike) : Logic  Inputs=3  AllPortsSameDT=off  OutDataTypeStr=boolean
  and11 : Logic  Operator=OR  Inputs=3  AllPortsSameDT=off  OutDataTypeStr=boolean
  and{4..5,8,13,16,19,21,23..26} (11 alike) : Logic  AllPortsSameDT=off  OutDataTypeStr=boolean
  and{2,6,9,14,17,20,22} (7 alike) : Logic  Operator=OR  AllPortsSameDT=off  OutDataTypeStr=boolean
  or1 : Logic  Operator=OR  Inputs=3  AllPortsSameDT=off  OutDataTypeStr=boolean
  or{2,4..19} (17 alike) : Logic  Operator=NOT  Inputs=1  AllPortsSameDT=off  OutDataTypeStr=boolean
  or3 : Logic  Operator=OR  AllPortsSameDT=off  OutDataTypeStr=boolean
  "primaryJetCommand " : Outport
  wires:
  rotationCommand/1 -> For Iterator Subsystem/2(rotationCommand)
  compensationCommand/1 -> For Iterator Subsystem/1(compensationCommand)
  PITCH_HI_LOW_SW/1 -> HI_PITCH/1
  NO_PLUS_Z_JETS/1 -> HI_PITCH/2, [NO_PLUS_Z_JETS]
  PITCH_TAIL_NOSE_SW/1 -> or1/3
  For Iterator Subsystem/1(bitCommand) -> [bitCommand]
  [bitCommand] -> Selector/1
  Selector/1 -> or1/1
  or1/1 -> NOSE_PITCH/1
  NOSE_PITCH/1 -> [NOSE_PITCH], or3/2
  HI_PITCH/1 -> or1/2, or3/1
  or3/1 -> and1/3, and/3  "C11"
  Selector1/1 -> and/1
  [bitCommand] -> Selector1/1
  [bitCommand] -> Selector2/1
  Selector2/1 -> and/2
  or4/1 -> and/4
  [NO_PLUS_Z_JETS] -> or4/1
  and/1 -> Mux/1
  Selector3/1 -> or5/1
  [bitCommand] -> Selector3/1
  or5/1 -> and1/1
  [bitCommand] -> Selector4/1
  Selector4/1 -> and1/2
  and1/1 -> Mux/3, Mux/2
  [bitCommand] -> Selector6/1, Selector5/1
  Selector5/1 -> or6/1
  Selector6/1 -> or2/1
  Selector7/1 -> or7/1
  [bitCommand] -> Selector8/1, Selector9/1, Selector7/1
  or7/1 -> and3/1
  Selector8/1 -> and3/3
  Selector9/1 -> or8/1
  or8/1 -> and3/2
  or9/1 -> and4/1
  [NOSE_PITCH] -> or9/1
  [NO_PLUS_Z_JETS] -> or10/1
  or10/1 -> and4/2
  and4/1 -> and8/2, and5/2  "C32"
  and6/1 -> and5/1
  and3/1 -> and9/2, and6/2  "C22"
  and7/1 -> and6/1
  and2/1 -> and10/3, and7/3  "C12"
  [bitCommand] -> Selector11/1, Selector10/1
  Selector10/1 -> and7/1
  Selector11/1 -> and7/2
  and5/1 -> Mux/4
  and8/1 -> Mux/5
  and9/1 -> and8/1
  and10/1 -> and9/1
  Selector12/1 -> or11/1
  [bitCommand] -> Selector12/1
  or11/1 -> and10/1
  Selector13/1 -> and10/2
  [bitCommand] -> Selector13/1
  Selector16/1 -> and11/2
  and11/1 -> and18/3, and15/3  "C13"
  or12/1 -> and11/3
  [bitCommand] -> Selector14/1, Selector16/1
  Selector14/1 -> or12/1
  [NO_PLUS_Z_JETS] -> and11/1
  Selector18/1 -> and12/2
  or13/1 -> and12/1
  Selector15/1 -> or13/1
  Selector17/1 -> and12/3
  [bitCommand] -> Selector17/1, Selector18/1, Selector15/1
  or14/1 -> and13/2
  [NOSE_PITCH] -> or14/1
  and14/1 -> and13/1
  and12/1 -> and17/2, and14/2
  or15/1 -> and15/1
  Selector20/1 -> and15/2
  [bitCommand] -> Selector20/1
  Selector19/1 -> or15/1
  [bitCommand] -> Selector19/1
  and15/1 -> and14/1
  and13/1 -> Mux/6
  [NOSE_PITCH] -> or16/1
  or16/1 -> and16/2
  and16/1 -> Mux/7
  and17/1 -> and16/1
  and18/1 -> and17/1
  [bitCommand] -> Selector22/1
  [bitCommand] -> Selector21/1
  Selector22/1 -> and18/2
  Selector21/1 -> and18/1
  and20/1 -> and19/1
  [bitCommand] -> Selector23/1
  Selector23/1 -> and19/2
  or17/1 -> and20/2
  and22/1 -> and21/1
  Selector24/1 -> and21/2
  YAW_TAIL_NOSE_SW/1 -> and22/2, or17/1
  YAW_HI_LOW_SW/1 -> and22/1, and20/1
  [bitCommand] -> Selector24/1
  or18/1 -> and23/1
  Selector25/1 -> or18/1
  [bitCommand] -> Selector25/1
  Selector26/1 -> and24/1
  [bitCommand] -> Selector26/1
  and19/1 -> and24/2, and23/2
  and23/1 -> Mux/8
  and24/1 -> Mux/9
  [bitCommand] -> Selector27/1
  and25/1 -> Mux/10
  Selector27/1 -> and25/1
  and21/1 -> and26/2, and25/2
  or19/1 -> and26/1
  Selector28/1 -> or19/1
  [bitCommand] -> Selector28/1
  and26/1 -> Mux/11
  Mux/1 -> "primaryJetCommand "/1
  or6/1 -> and2/1
  or2/1 -> and2/2
